simulink model "RRRsimulationwentaoxu"  (R2017a)
settings: Solver=VariableStepAuto  StartTime=0.0  StopTime=10  RelTol=1e-3
settings Model: Creator=lenovo  LastModifiedBy=lenovo

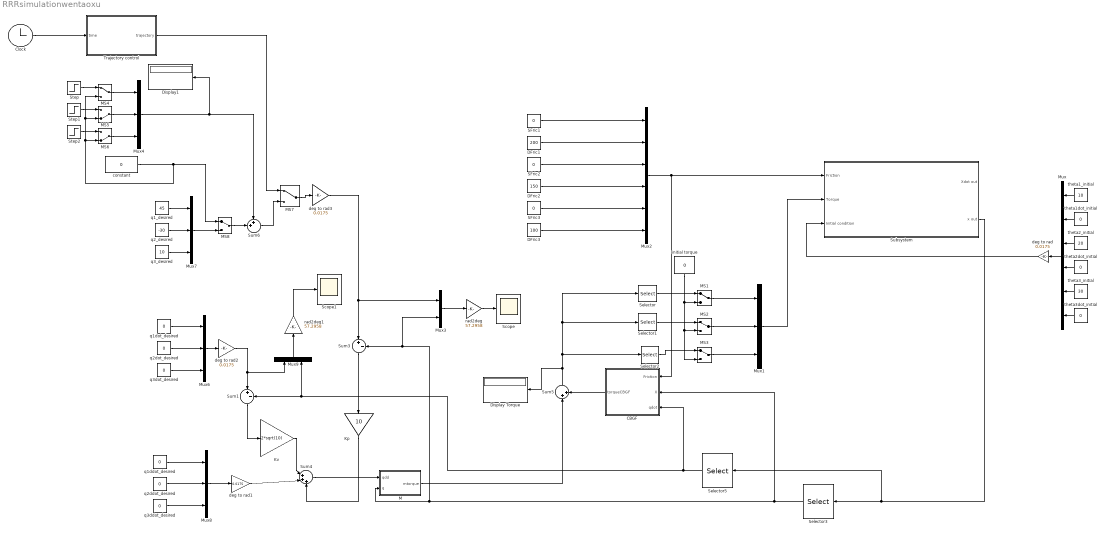
== system RRRsimulationwentaoxu ==
  "CBGF " : MATLAB Function  TreatAsAtomicUnit=on
  Clock : Clock
      settings: Decimation=100
  DFric1 : Constant  Value=200
  DFric2 : Constant  Value=150
  DFric3 : Constant  Value=100
  Display Torque : Display
  Display1 : Display
  Kp : Gain  Gain=10
  Kv : Gain  Gain=2*sqrt(10)
  M : MATLAB Function  TreatAsAtomicUnit=on
  MS{1..4,7..8} (6 alike) : ManualSwitch
  MS5 : ManualSwitch  CurrentSetting=0
  MS6 : ManualSwitch  CurrentSetting=0
  Mux : Mux  Inputs=6
  Mux{1,4,6..8} (5 alike) : Mux  Inputs=3
  Mux2 : Mux  Inputs=6
  Mux3 : Mux  Inputs=2
  Mux9 : Mux  Inputs=2
  SFric1 : Constant  Value=0
  SFric2 : Constant  Value=0
  SFric3 : Constant  Value=0
  Scope : Scope
  Scope1 : Scope
  Selector : Selector  InputPortWidth=3  IndexOptions=Index vector (dialog)  Indices=[1]  OutputSizes=1
  Selector1 : Selector  InputPortWidth=3  IndexOptions=Index vector (dialog)  Indices=[2]  OutputSizes=1
  Selector2 : Selector  InputPortWidth=3  IndexOptions=Index vector (dialog)  Indices=[3]  OutputSizes=1
  Selector3 : Selector  InputPortWidth=6  IndexOptions=Index vector (dialog)  Indices=[1 3 5]  OutputSizes=1
  Selector5 : Selector  InputPortWidth=6  IndexOptions=Index vector (dialog)  Indices=[2 4 6]  OutputSizes=1
  Step : Step  Time=0  After=45  SampleTime=0
  Step1 : Step  Time=0  SampleTime=0
  Step2 : Step  Time=0  SampleTime=0
  Subsystem : Subsystem
  Sum1 : Sum  Inputs=|+-
  Sum3 : Sum  Inputs=|+-
  Sum4 : Sum  Inputs=|+++
  Sum5 : Sum  Inputs=|++
  Sum6 : Sum  Inputs=++|
  Trajectory control : MATLAB Function  TreatAsAtomicUnit=on
  constant : Constant  Value=0
  deg to rad{,1..3} (4 alike) : Gain  Gain=0.0175
  initial torque : Constant  Value=0
  q1_desired : Constant  Value=45
  q1ddot_desired : Constant  Value=0
  q1dot_desired : Constant  Value=0
  q2_desired : Constant  Value=-30
  q2ddot_desired : Constant  Value=0
  q2dot_desired : Constant  Value=0
  q3_desired : Constant  Value=10
  q3ddot_desired : Constant  Value=0
  q3dot_desired : Constant  Value=0
  rad2deg : Gain  Gain=57.2958
  rad2deg1 : Gain  Gain=57.2958
  theta1_initial : Constant  Value=10
  theta1dot_initial : Constant  Value=0
  theta2_initial : Constant  Value=20
  theta2dot_initial : Constant  Value=0
  theta3_initial : Constant  Value=30
  theta3dot_initial : Constant  Value=0
  wires:
  DFric3/1 -> Mux2/6
  SFric3/1 -> Mux2/5
  DFric1/1 -> Mux2/2
  SFric1/1 -> Mux2/1
  SFric2/1 -> Mux2/3
  DFric2/1 -> Mux2/4
  Mux2/1 -> "CBGF "/1(Friction), Subsystem/1(Friction)
  theta3_initial/1 -> Mux/5
  theta3dot_initial/1 -> Mux/6
  theta2dot_initial/1 -> Mux/4
  theta1dot_initial/1 -> Mux/2
  theta2_initial/1 -> Mux/3
  theta1_initial/1 -> Mux/1
  Mux/1 -> deg to rad/1
  deg to rad/1 -> Subsystem/3(Initial condition)
  Subsystem/2(x out) -> Selector3/1, Selector5/1
  Mux1/1 -> Subsystem/2(Torque)
  Selector/1 -> MS1/1
  MS1/1 -> Mux1/1
  MS2/1 -> Mux1/2
  Selector1/1 -> MS2/1
  MS3/1 -> Mux1/3
  Selector2/1 -> MS3/1
  initial torque/1 -> MS1/2, MS2/2, MS3/2
  q3dot_desired/1 -> Mux6/3
  q3_desired/1 -> Mux7/3
  q1_desired/1 -> Mux7/1
  q2_desired/1 -> Mux7/2
  q2dot_desired/1 -> Mux6/2
  q1dot_desired/1 -> Mux6/1
  q1ddot_desired/1 -> Mux8/1
  q2ddot_desired/1 -> Mux8/2
  q3ddot_desired/1 -> Mux8/3
  Mux8/1 -> deg to rad1/1
  Mux6/1 -> deg to rad2/1
  deg to rad2/1 -> Mux9/1, Sum1/1
  Sum1/1 -> Kv/1
  Selector3/1 -> Mux3/2, Sum3/2, M/2(q), "CBGF "/2(X)
  Kv/1 -> Sum4/1
  Selector5/1 -> Mux9/2, Sum1/2, "CBGF "/3(qdot)
  Mux3/1 -> rad2deg/1
  rad2deg/1 -> Scope/1
  rad2deg1/1 -> Scope1/1
  Mux9/1 -> rad2deg1/1
  Sum4/1 -> M/1(qdd)
  M/1(mtorque) -> Sum5/1
  "CBGF "/1(torqueCBGF) -> Sum5/2
  Sum5/1 -> Display Torque/1, Selector2/1, Selector1/1, Selector/1
  deg to rad3/1 -> Mux3/1, Sum3/1
  Sum3/1 -> Kp/1
  Kp/1 -> Sum4/3
  Step/1 -> MS4/1
  Step2/1 -> MS6/1
  constant/1 -> MS6/2, MS4/2, MS5/2, MS8/1
  Step1/1 -> MS5/1
  MS4/1 -> Mux4/1
  MS6/1 -> Mux4/3
  MS5/1 -> Mux4/2
  Clock/1 -> Trajectory control/1(time)
  Sum6/1 -> MS7/2
  MS7/1 -> deg to rad3/1
  Trajectory control/1(trajectory) -> MS7/1
  MS8/1 -> Sum6/2
  Mux7/1 -> MS8/2
  Mux4/1 -> Display1/1, Sum6/1
  deg to rad1/1 -> Sum4/2

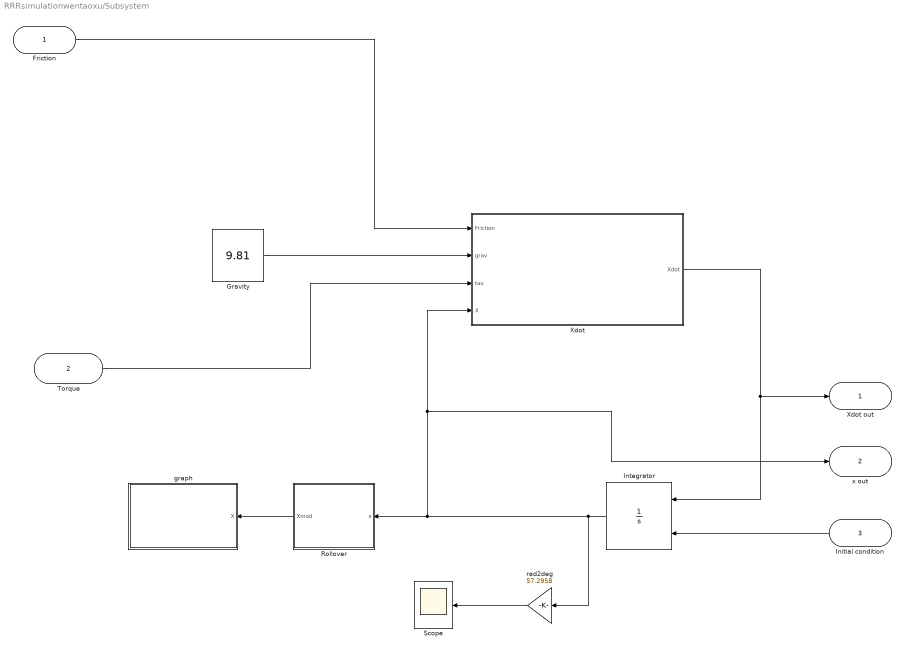
== system RRRsimulationwentaoxu/Subsystem ==
  Friction : Inport
  Torque : Inport  Port=2
  Initial condition : Inport  Port=3
  Gravity : Constant  Value=9.81
  Integrator : Integrator  InitialConditionSource=external
  Rollover : MATLAB Function  TreatAsAtomicUnit=on
  Scope : Scope
  Xdot : MATLAB Function  TreatAsAtomicUnit=on
  graph : MATLAB Function  TreatAsAtomicUnit=on
  rad2deg : Gain  Gain=57.2958
  Xdot out : Outport
  x out : Outport  Port=2
  wires:
  Gravity/1 -> Xdot/2(grav)
  Integrator/1 -> rad2deg/1, Rollover/1(x), x out/1, Xdot/4(X)
  Xdot/1(Xdot) -> Xdot out/1, Integrator/1
  rad2deg/1 -> Scope/1
  Friction/1 -> Xdot/1(Friction)
  Initial condition/1 -> Integrator/2
  Torque/1 -> Xdot/3(tau)
  Rollover/1(Xmod) -> graph/1(X)

== matlab function RRRsimulationwentaoxu/Subsystem/graph ==
  data: X input
function RRRgraphsimulator(X)
L1=4;
L2=3;
L3=2;
q1=X(1);
q2=X(3);
q3=X(5);
P1=[L1;0;0;1];
P2=[L2;0;0;1];
P3=[L3;0;0;1];
c1=cos(q1);
c2=cos(q2);
c3=cos(q3);
s1=sin(q1);
s2=sin(q2);
s3=sin(q3);
T01=[c1 -s1 0 0; s1 c1 0 0; 0 0 1 0; 0 0 0 1];
T12=[c2 -s2 0 L1; s2 c2 0 0; 0 0 1 0; 0 0 0 1];
T23=[c3 -s3 0 L2; s3 c3 0 0; 0 0 1 0; 0 0 0 1];
T02=T01*T12;
T03=T02*T23;
arm1=T01*P1;
arm2=T02*P2;
arm3=T03*P3;
joint1 = [0;0];
joint2 = [arm1(1);arm1(2)];
joint3 = [arm2(1);arm2(2)];
joint4 = [arm3(1);arm3(2)];
hold off
plot([joint2(1);joint1(1)],[joint2(2);joint1(2)],'r','LineWidth',3);hold on
plot([joint3(1);joint2(1)],[joint3(2);joint2(2)],'y','LineWidth',3);hold on
plot([joint4(1);joint3(1)],[joint4(2);joint3(2)],'b','LineWidth',2);hold on
plot(joint1(1),joint1(2),'ko',joint2(1),joint2(2),'ko',joint3(1),joint3(2),'ko',joint4(1),joint4(2),'ko');hold on
title('RRR Robotic Arm Simulator'), xlabel('X'), ylabel('Y');grid on
axis([-10, 10, -10, 10]);
end

== matlab function RRRsimulationwentaoxu/Subsystem/Xdot ==
  data: Friction input; grav input; tau input; X input; Xdot output
function Xdot  = Xdot(Friction,grav,tau,X)
q1=X(1);
q1dot=X(2);
q2=X(3);
q2dot=X(4);
q3=X(5);
q3dot=X(6);
torque1=tau(1);
torque2=tau(2);
torque3=tau(3);

SFric1=Friction(1);
DFric1=Friction(2);
SFric2=Friction(3);
DFric2=Friction(4);
SFric3=Friction(5);
DFric3=Friction(6);
Frc1=SFric1*sign(q1dot) + DFric1*q1dot;
Fric2=SFric2*sign(q2dot) + DFric2*q2dot;
Fric3=SFric3*sign(q3dot) + DFric3*q3dot;
Friction=[Frc1;Fric2;Fric3];

MassMatrix=zeros(3);
MassMatrix(1,1)=80*cos(q2+q3)+420*cos(q2)+60*cos(q3)+12291/20;
MassMatrix(1,2)=40*cos(q2+q3)+210*cos(q2)+60*cos(q3)+2681/20;
MassMatrix(1,3)=40*cos(q2+q3)+30*cos(q3)+101/10;
MassMatrix(2,1)=40*cos(q2+q3)+210*cos(q2)+60*cos(q3)+2681/20;
MassMatrix(2,2)=60*cos(q3)+2681*20;
MassMatrix(2,3)=30*cos(q3)+101/10;
MassMatrix(3,1)=40*cos(q2+q3)+30*cos(q3)+101/10;
MassMatrix(3,2)=30*cos(q3)+101/10;
MassMatrix(3,3)=101/10;
CMatrix=zeros(3);
CMatrix(1,2)=-40*sin(q2+q3)-210*sin(q2);
CMatrix(1,3)=-40*sin(q2+q3)-30*sin(q3);
CMatrix(2,1)=40*sin(q2+q3)+210*sin(q2);
CMatrix(2,3)=-30*sin(q3);
CMatrix(3,1)=40*sin(q2+q3)+30*sin(q3);
CMatrix(3,2)=30*sin(q3);
BMatrix=zeros(3);
BMatrix(1,1)=-80*sin(q2+q3)-420*sin(q2);
BMatrix(1,2)=-80*sin(q2+q3)-60*sin(q3);
BMatrix(1,3)=-80*sin(q2+q3)-60*sin(q3);
BMatrix(2,2)=-60*sin(q3);
BMatrix(2,3)=-60*sin(q3);
BMatrix(3,1)=60*sin(q3);
GMatrix=zeros(3,1);
GMatrix(1)=15*grav*(3*cos(q1+q2)/2+4*cos(q1)) + 10*grav*(cos(q1+q2+q3) + 3*cos(q1+q2) + 4*cos(q1)) + 40*grav*cos(q1);
GMatrix(2)=10*grav*(cos(q1+q2+q3) + 3*cos(q1+q2)) + (45*grav*cos(q1+q2))/2;
GMatrix(3)=10*grav*cos(q1+q2+q3);

qdd=MassMatrix\([torque1;torque2;torque3] - CMatrix*[q1dot^2;q2dot^2;q3dot^2] - BMatrix*[q1dot*q2dot;q1dot*q3dot;q2dot*q3dot] - GMatrix - Friction );

Xdot=zeros(6,1);
Xdot(1)=q1dot;
Xdot(2)=qdd(1);
Xdot(3)=q2dot;
Xdot(4)=qdd(2);
Xdot(5)=q3dot;
Xdot(6)=qdd(3);
end

== matlab function RRRsimulationwentaoxu/CBGF  ==
  data: Friction input; torqueCBGF output; X input; qdot input
function torqueCBGF= fcn(Friction,X,qdot)
grav=9.81;
q1=X(1);
q2=X(2);
q3=X(3);
q1dot=qdot(1);
q2dot=qdot(2);
q3dot=qdot(3);
SFric1=Friction(1);
DFric1=Friction(2);
SFric2=Friction(3);
DFric2=Friction(4);
SFric3=Friction(5);
DFric3=Friction(6);
fric1=SFric1*sign(q1dot) + DFric1*q1dot;
fric2=SFric2*sign(q2dot) + DFric2*q2dot;
fric3=SFric3*sign(q3dot) + DFric3*q3dot;
Friction=[fric1;fric2;fric3];


CMatrix=zeros(3,3);
CMatrix(1,2)=-40*sin(q2+q3)-210*sin(q2);
CMatrix(1,3)=-40*sin(q2+q3)-30*sin(q3);
CMatrix(2,1)=40*sin(q2+q3)+210*sin(q2);
CMatrix(2,3)=-30*sin(q3);
CMatrix(3,1)=40*sin(q2+q3)+30*sin(q3);
CMatrix(3,2)=30*sin(q3);

BMatrix=zeros(3,3);
BMatrix(1,1)=-80*sin(q2+q3)-420*sin(q2);
BMatrix(1,2)=-80*sin(q2+q3)-60*sin(q3);
BMatrix(1,3)=-80*sin(q2+q3)-60*sin(q3);
BMatrix(2,2)=-60*sin(q3);
BMatrix(2,3)=-60*sin(q3);
BMatrix(3,1)=60*sin(q3);

GMatrix=zeros(3,1);
GMatrix(1)=15*grav*(3*cos(q1+q2)/2+4*cos(q1)) + 10*grav*(cos(q1+q2+q3) + 3*cos(q1+q2) + 4*cos(q1)) + 40*grav*cos(q1);
GMatrix(2)=10*grav*(cos(q1+q2+q3) + 3*cos(q1+q2)) + (45*grav*cos(q1+q2))/2;
GMatrix(3)=10*grav*cos(q1+q2+q3);

torqueCBGF = CMatrix*[q1dot^2;q2dot^2;q3dot^2] + BMatrix*[q1dot*q2dot;q1dot*q3dot;q2dot*q3dot] + GMatrix + Friction;
end

== matlab function RRRsimulationwentaoxu/Subsystem/Rollover ==
  data: x input; Xmod output
function Xmod = fcn(x)
q1=x(1);
q2=x(3);
q3=x(5);
q1=atan2(sin(q1),cos(q1));
q2=atan2(sin(q2),cos(q2));
q3=atan2(sin(q3),cos(q3));
Xmod = [q1;x(2);q2;x(4);q3;x(6)];

== matlab function RRRsimulationwentaoxu/M ==
  data: qdd input; q input; mtorque output
function mtorque = Mass(qdd,q)
q2=q(2);
q3=q(3);
MassMatrix=zeros(3,3);
MassMatrix(1,1)=80*cos(q2+q3)+420*cos(q2)+60*cos(q3)+12291/20;
MassMatrix(1,2)=40*cos(q2+q3)+210*cos(q2)+60*cos(q3)+2681/20;
MassMatrix(1,3)=40*cos(q2+q3)+30*cos(q3)+101/10;
MassMatrix(2,1)=40*cos(q2+q3)+210*cos(q2)+60*cos(q3)+2681/20;
MassMatrix(2,2)=60*cos(q3)+2681*20;
MassMatrix(2,3)=30*cos(q3)+101/10;
MassMatrix(3,1)=40*cos(q2+q3)+30*cos(q3)+101/10;
MassMatrix(3,2)=30*cos(q3)+101/10;
MassMatrix(3,3)=101/10;
mtorque=MassMatrix*[qdd(1);qdd(2);qdd(3)];
end

== matlab function RRRsimulationwentaoxu/Trajectory control ==
  data: time input; trajectory output
function trajectory = Trajectroy(time)
Time_angletable_initialvalue=[0,0,0,90;2,30,-10,70;4,45,130,-85;6,150,10,70;8,180,0,-90];
T1=Time_angletable_initialvalue(:,1);
T2=Time_angletable_initialvalue(:,2)';
T3=Time_angletable_initialvalue(:,3)';
T4=Time_angletable_initialvalue(:,4)';
q1=spline(T1,[0, T2, 0]);
q2=spline(T1,[0, T3, 0]);
q3=spline(T1,[0, T4, 0]);
Ts=0:.01:8;
table=[Ts',ppval(q1,Ts)',ppval(q2,Ts)',ppval(q3,Ts)'];
% plot(T1,T2,'o',Ts,ppval(q1,Ts),'-');hold on
% plot(T1,T3,'o',Ts,ppval(q2,Ts),'-');hold on
% plot(T1,T4,'o',Ts,ppval(q3,Ts),'-');hold on
[~, idx] = min(abs(time-table(:,1)));
trajectory= table(idx,2:4)';
end
